simulink model "testing"  (R2018b)
settings: Solver=FixedStepDiscrete  StartTime=0.0  StopTime=inf  FixedStep=1/400  RelTol=1e-3
values from neighbouring files (symbols this model uses):
  conf = Configuration    [config.m]
libraries: libslotcar x3, simulink x1, sldrtlib x1
settings Model: Creator=petrb  LastModifiedBy=Lenovo
settings SolverCC: PositivePriorityOrder=on
settings OptimizationCC: PassReuseOutputArgsAs=Individual arguments  MaxStackSize=64
settings DebuggingCC: ParameterTunabilityLossMsg=error  LibraryContextMissingDiagnostic=none
settings HardwareCC: ProdBitPerPointer=32  ProdBitPerSizeT=32  ProdBitPerPtrDiffT=32  ProdLargestAtomicInteger=Long  ProdLargestAtomicFloat=Double  ProdWordSize=32  ProdHWDeviceType=ARM Compatible->ARM Cortex
settings SFSimCC: SimUseLocalCustomCode=off  MATLABDynamicMemAlloc=off
settings RTWCC: SystemTargetFile=ert.tlc  HardwareBoard=BeagleBone Blue  TLCOptions="-aInlineSetEventsForThisBaseRateFcn=TLC_FALSE -aSuppressMultiTaskScheduler=TLC_FALSE  -aRateBasedStepFcn=0"  TemplateMakefile=ert_default_tmf  RTWUseLocalCustomCode=off  RTWUseSimCustomCode=on  Toolchain=GNU GCC BeagleBone Blue  IncludeHyperlinkInReport=on
settings CodeAppCC: ForceParamTrailComments=on  IgnoreCustomStorageClasses=off  OperatorAnnotations=on  SimulinkDataObjDesc=on  SFDataObjDesc=on  InsertBlockDesc=on
settings ERTTargetCC: SupportNonInlinedSFcns=on  SupportVariableSizeSignals=on

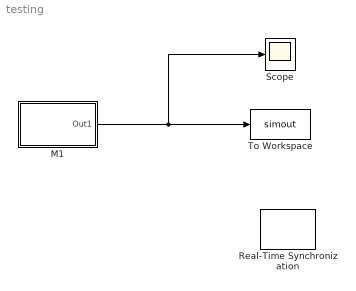
== system testing ==
  M1 : Subsystem
  Real-Time Synchronization : sldrtlib/Real-Time Synchronization  SampleTime=conf.CommsBackend.SampleTime  MaxMissedTicks=40402  ShowMissedTicks=off  YieldWhenWaiting=on
  Scope : Scope
  To Workspace : ToWorkspace  VariableName=simout  SaveFormat=Timeseries  SampleTime=-1
  wires:
  M1/1(Out1) -> Scope/1, To Workspace/1

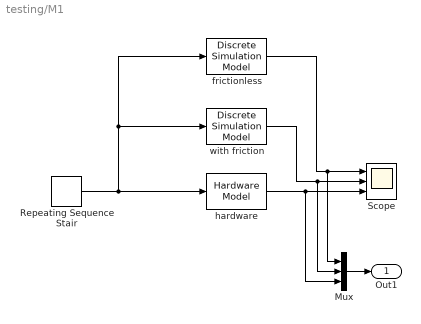
== system testing/M1 ==
  Mux : Mux  Inputs=3
  Repeating Sequence Stair : simulink/Sources/Repeating Sequence Stair  OutValues=[.3 .35 .4 .2 .25].'  tsamp=2  OutMin=[]  OutMax=[]  OutDataTypeStr=double  OutputDataTypeScalingMode=double  OutDataType=fixdt(0,8)  ConRadixGroup=Best Precision: Vector-wise  OutScaling=2^-12
  Scope : Scope  NumInputPorts=3
  frictionless : libslotcar/Discrete Simulation Model  tsparam=1/400  mparam=0.17733  dparam=0.018  nparam=9/28  uparam=12.25-0.7  rparam=5  kparam=0.005  ksparam=0  kdparam=0
  hardware : libslotcar/Hardware Model  freq=25000  SampleTime=1/400  encts=1/50  encres=20  gearratio=9/28  diameter=0.018  reversed=on
  with friction : libslotcar/Discrete Simulation Model  tsparam=1/400  mparam=0.17733  dparam=0.018  nparam=9/28  uparam=12.25-0.7  rparam=5  kparam=0.005  ksparam=0.6739  kdparam=0.3317
  Out1 : Outport
  wires:
  Repeating Sequence Stair/1 -> hardware/1, frictionless/1, with friction/1
  Mux/1 -> Out1/1
  frictionless/1 -> Mux/1, Scope/1
  with friction/1 -> Mux/2, Scope/2
  hardware/1 -> Mux/3, Scope/3
